simulink model "M1_P3_A_4"  (R2023a)
settings: Solver=VariableStepAuto  StartTime=0.0  StopTime=10  RelTol=1e-3
undefined symbols (not defined in the file): f_eff, J_eff, Kb, Ktn, L, R
settings Model: Creator=azzam  LastModifiedBy=azzam

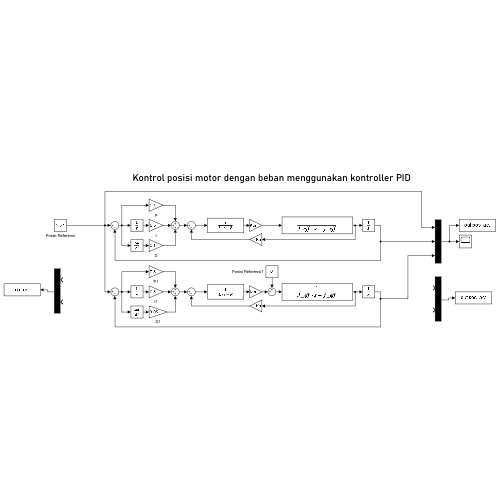
[thumbnail: Simulink's stored preview of the top-level diagram]
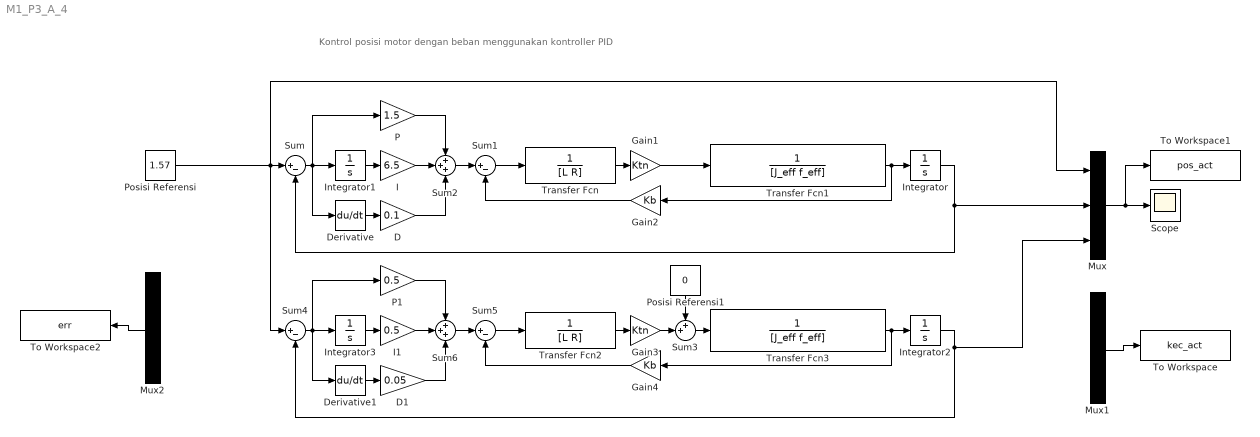
== system M1_P3_A_4 ==
  note: Kontrol posisi motor dengan beban menggunakan kontroller PID
  D : Gain  Gain=0.1
  D1 : Gain  Gain=0.05
  Derivative : Derivative
  Derivative1 : Derivative
  Gain1 : Gain  Gain=Ktn
  Gain2 : Gain  Gain=Kb
  Gain3 : Gain  Gain=Ktn
  Gain4 : Gain  Gain=Kb
  I : Gain  Gain=6.5
  I1 : Gain  Gain=0.5
  Integrator{,1..3} (4 alike) : Integrator
  Mux : Mux  Inputs=3
  Mux1 : Mux  Inputs=2
  Mux2 : Mux  Inputs=2
  P : Gain  Gain=1.5
  P1 : Gain  Gain=0.5
  Posisi Referensi : Constant  Value=1.57
  Posisi Referensi1 : Constant  Value=0
  Scope : Scope
  Sum{,1,4..5} (4 alike) : Sum  Inputs=|+-
  Sum2 : Sum  Inputs=+++
  Sum3 : Sum  Inputs=++|
  Sum6 : Sum  Inputs=+++
  To Workspace : ToWorkspace  VariableName=kec_act  SaveFormat=Timeseries  SampleTime=-1
  To Workspace1 : ToWorkspace  VariableName=pos_act  SaveFormat=Timeseries  SampleTime=-1
  To Workspace2 : ToWorkspace  VariableName=err  SaveFormat=Timeseries  SampleTime=-1
  Transfer Fcn : TransferFcn  Denominator=[L R]
  Transfer Fcn1 : TransferFcn  Denominator=[J_eff f_eff]
  Transfer Fcn2 : TransferFcn  Denominator=[L R]
  Transfer Fcn3 : TransferFcn  Denominator=[J_eff f_eff]
  wires:
  Transfer Fcn/1 -> Gain1/1
  Transfer Fcn1/1 -> Gain2/1, Integrator/1
  Sum2/1 -> Sum1/1
  Sum1/1 -> Transfer Fcn/1
  D/1 -> Sum2/3
  Mux/1 -> To Workspace1/1, Scope/1
  P/1 -> Sum2/1
  Derivative/1 -> D/1
  Mux2/1 -> To Workspace2/1
  Integrator/1 -> Mux/2, Sum/2
  Gain2/1 -> Sum1/2
  Sum/1 -> Integrator1/1, Derivative/1, P/1
  Mux1/1 -> To Workspace/1
  Integrator1/1 -> I/1
  I/1 -> Sum2/2
  Posisi Referensi/1 -> Sum4/1, Mux/1, Sum/1
  Integrator3/1 -> I1/1
  Sum5/1 -> Transfer Fcn2/1
  Transfer Fcn2/1 -> Gain3/1
  I1/1 -> Sum6/2
  Sum4/1 -> Integrator3/1, Derivative1/1, P1/1
  Derivative1/1 -> D1/1
  P1/1 -> Sum6/1
  Sum6/1 -> Sum5/1
  D1/1 -> Sum6/3
  Gain4/1 -> Sum5/2
  Integrator2/1 -> Mux/3, Sum4/2
  Transfer Fcn3/1 -> Gain4/1, Integrator2/1
  Gain1/1 -> Transfer Fcn1/1
  Gain3/1 -> Sum3/2
  Sum3/1 -> Transfer Fcn3/1
  Posisi Referensi1/1 -> Sum3/1
